simulink model "no4_PID_Controller_22b"  (R2022b)
settings: Solver=VariableStepAuto  StartTime=0.0  StopTime=50  RelTol=1e-3
libraries: simulink x1
settings Model: Creator=ayeo  LastModifiedBy=ayeo
settings OptimizationCC: ReuseModelBlockBuffer=on
settings RTWCC: GPUComputeCapability=5.0
settings ConfigComp: CovBoundaryAbsTol=1.0e-5

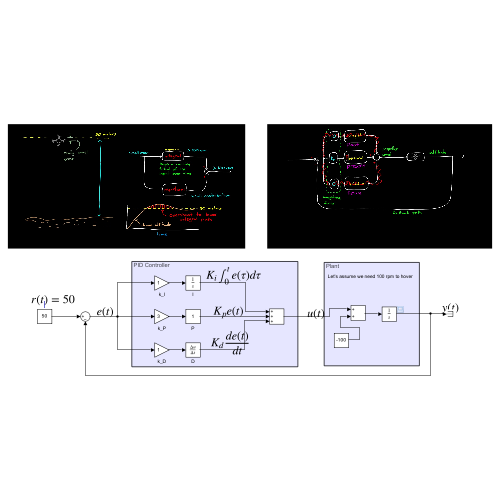
[thumbnail: Simulink's stored preview of the top-level diagram]
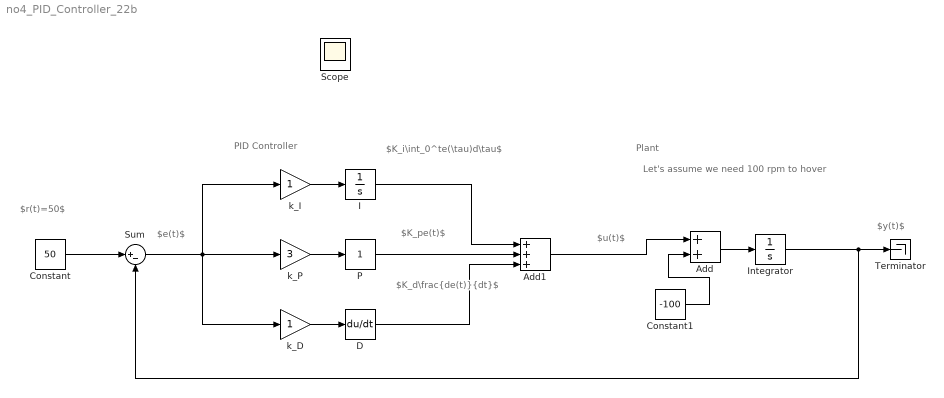
== system no4_PID_Controller_22b ==
  note: Plant
  note: $K_pe(t)$
  note: PID Controller
  note: Let's assume we need 100 rpm to hover
  note: $K_i\int_0^te(\tau)d\tau$
  note: $K_d\frac{de(t)}{dt}$
  note: $r(t)=50$
  note: $u(t)$
  note: $y(t)$
  note: $e(t)$
  Add : Sum
  Add1 : Sum  Inputs=+++
  Constant : Constant  Value=50
  Constant1 : Constant  Value=-100
  D : Derivative  CoefficientInTFapproximation=Inf
  I : Integrator
  Integrator : Integrator
  P : simulink/Math Operations/Slider Gain  gain=1  low=0.1  high=100
  Sum : Sum  Inputs=|+-
  Terminator : Terminator
  k_D : Gain
  k_I : Gain
  k_P : Gain  Gain=3
  Scope : Scope
  wires:
  Constant/1 -> Sum/1
  Integrator/1 -> Sum/2, Terminator/1
  Add/1 -> Integrator/1
  Constant1/1 -> Add/2
  Add1/1 -> Add/1
  k_D/1 -> D/1
  k_P/1 -> P/1
  k_I/1 -> I/1
  D/1 -> Add1/3
  Sum/1 -> k_P/1, k_D/1, k_I/1
  I/1 -> Add1/1
  P/1 -> Add1/2
